simulink model "RefModel_FlightPerf"  (R2020a)
settings: Solver=ode1  StartTime=0.0  StopTime=10.0  FixedStep=Ts_Task.Ts_base  RelTol=1e-3
values from neighbouring files (symbols this model uses):
  TaskParam = TASK_SET.PathPlanner    [INIT_TASK.m]
undefined symbols (not defined in the file or in its folder): FlightPerfParam
settings Model: Creator=sl  LastModifiedBy=sl
settings DataIOCC: SaveOutput=off  SaveTime=off
settings OptimizationCC: DefaultParameterBehavior=Inlined  EnhancedBackFolding=on  PassReuseOutputArgsAs=Individual arguments  ZeroExternalMemoryAtStartup=off  ZeroInternalMemoryAtStartup=off  OptimizeBlockOrder=speed  DifferentSizesBufferReuse=on  OptimizationCustomize=off  EfficientTunableParamExpr=on
settings DebuggingCC: InheritedTsInSrcMsg=none  ParameterPrecisionLossMsg=none  ParameterTunabilityLossMsg=error  UnconnectedInputMsg=none  UnconnectedOutputMsg=none  UnconnectedLineMsg=none
settings HardwareCC: ProdBitPerPointer=32  ProdBitPerSizeT=32  ProdBitPerPtrDiffT=32  ProdLargestAtomicInteger=Long  ProdLargestAtomicFloat=Double  ProdWordSize=32  ProdHWDeviceType=ARM Compatible->ARM Cortex
settings ModelReferenceCC: ModelReferenceNumInstancesAllowed=Single  PropagateVarSize=During execution
settings SFSimCC: MATLABDynamicMemAlloc=off
settings RTWCC: SystemTargetFile=ert.tlc  TemplateMakefile=ert_default_tmf  GenerateReport=on  IncludeHyperlinkInReport=on  LaunchReport=on  GenerateTraceInfo=on  GenerateTraceReport=on  GenerateTraceReportSl=on  GenerateTraceReportSf=on  GenerateTraceReportEml=on
settings CodeAppCC: ForceParamTrailComments=on  IgnoreCustomStorageClasses=off  MaxIdLength=48  OperatorAnnotations=on  SimulinkDataObjDesc=on  SFDataObjDesc=on  MATLABFcnDesc=on  InsertBlockDesc=on  StateflowObjectComments=on  MATLABSourceComments=on
settings ERTTargetCC: TargetLangStandard=C99 (ISO)  GenerateSampleERTMain=on  LogVarNameModifier=none  SupportVariableSizeSignals=on  InlinedParameterPlacement=NonHierarchical  ERTCustomFileTemplate=example_file_process.tlc

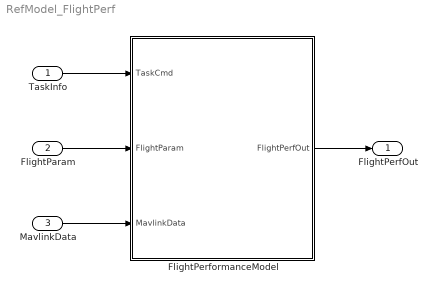
== system RefModel_FlightPerf ==
  TaskInfo : Inport  OutDataTypeStr=Bus: BUS_TASK_PATH_OutParam  BusOutputAsStruct=on
  FlightParam : Inport  Port=2  OutDataTypeStr=Bus: BUS_TASK_COMMON_OutParam  BusOutputAsStruct=on
  MavlinkData : Inport  Port=3  OutDataTypeStr=Bus: BUS_MAVLINK_TO_FIRM  PortDimensions=1  BusOutputAsStruct=on
  FlightPerformanceModel : Subsystem
  FlightPerfOut : Outport  OutDataTypeStr=Bus: BUS_FLIGHTPERF_OUT
  wires:
  MavlinkData/1 -> FlightPerformanceModel/3(MavlinkData)
  FlightPerformanceModel/1(FlightPerfOut) -> FlightPerfOut/1
  FlightParam/1 -> FlightPerformanceModel/2(FlightParam)
  TaskInfo/1 -> FlightPerformanceModel/1(TaskCmd)

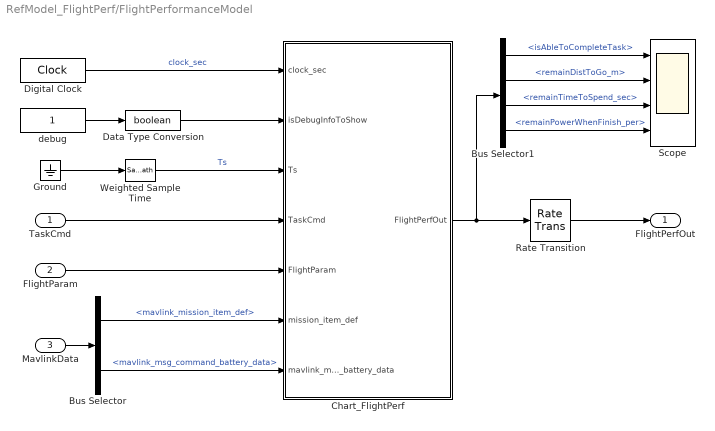
== system RefModel_FlightPerf/FlightPerformanceModel ==
  TaskCmd : Inport
  FlightParam : Inport  Port=2
  MavlinkData : Inport  Port=3
  Bus Selector : BusSelector  OutputSignals=mavlink_mission_item_def,mavlink_msg_command_battery_data
  Bus Selector1 : BusSelector  OutputSignals=isAbleToCompleteTask,remainDistToGo_m,remainTimeToSpend_sec,remainPowerWhenFinish_per
  Chart_FlightPerf : Stateflow chart  TreatAsAtomicUnit=on
  Data Type Conversion : DataTypeConversion  OutDataTypeStr=boolean
  Digital Clock : DigitalClock  SampleTime=-1
  Ground : Ground
  Rate Transition : RateTransition
  Scope : Scope  NumInputPorts=4
  Weighted Sample Time : SampleTimeMath  TsampMathOp=Ts Only
  debug : Constant
  FlightPerfOut : Outport
  wires:
  FlightParam/1 -> Chart_FlightPerf/5(FlightParam)
  debug/1 -> Data Type Conversion/1
  Data Type Conversion/1 -> Chart_FlightPerf/2(isDebugInfoToShow)
  Weighted Sample Time/1 -> Chart_FlightPerf/3(Ts)  "Ts"
  Digital Clock/1 -> Chart_FlightPerf/1(clock_sec)  "clock_sec"
  TaskCmd/1 -> Chart_FlightPerf/4(TaskCmd)
  MavlinkData/1 -> Bus Selector/1
  Ground/1 -> Weighted Sample Time/1
  Bus Selector/1 -> Chart_FlightPerf/6(mission_item_def)  "<mavlink_mission_item_def>"
  Chart_FlightPerf/1(FlightPerfOut) -> Bus Selector1/1, Rate Transition/1
  Bus Selector1/1 -> Scope/1  "<isAbleToCompleteTask>"
  Bus Selector1/2 -> Scope/2  "<remainDistToGo_m>"
  Bus Selector1/3 -> Scope/3  "<remainTimeToSpend_sec>"
  Bus Selector1/4 -> Scope/4  "<remainPowerWhenFinish_per>"
  Bus Selector/2 -> Chart_FlightPerf/7(mavlink_msg_command_battery_data)  "<mavlink_msg_command_battery_data>"
  Rate Transition/1 -> FlightPerfOut/1

== stateflow chart RefModel_FlightPerf/FlightPerformanceModel/Chart_FlightPerf ==
  state PowerConsumeByUavMode [parallel]
    settings: executionOrder=2
    state Rotor
      en:
    state Fix
      en:
    (default) -> PowerConsumeByUavMode.Rotor
    PowerConsumeByUavMode.Rotor -> Fix : [isUavInFix]
    Fix -> PowerConsumeByUavMode.Rotor : [isUavInRotor]
  state OverAllParam [parallel]
    settings: executionOrder=1
    state Rotor
      en:
      initFlightPerOut;
      du:
      on every(3,tick):
      predictDistToFly;
      on every(ceil(0.9/Ts),tick):
      predictTimeToFly;
      predictRemainPowerWhenComplete;
      isPowerEnoughToCompleteTask;
    (default) -> OverAllParam.Rotor
  data: flag function_output; debugInfo function_input; tabspace function_input; varargin function_input; flag function_output; modeName function_input; debugInfo function_input; varargin function_input; lla function_input; ll0 function_input; p function_output; clock_sec input; isDebugInfoToShow input; Ts input; TaskCmd input Bus: BUS_TASK_PATH_OutParam size=1; FlightParam input Bus: BUS_TASK_COMMON_OutParam size=1; mission_item_def input Bus: mavlink_mission_item_def size=TASK_SET.PathPlanner.maxPathPointNum; TaskParam parameter Bus: BUS_TASK_PATH_AlgoParam; FlightPerfParam parameter Bus: BUS_FLIGHTPERF_PARAM size=1; FlightPerfOut output Bus: BUS_FLIGHTPERF_OUT size=1; mavlink_msg_command_battery_data input Bus: mavlink_msg_command_battery_data size=1
  function predictRemainPowerWhenComplete:
    | function predictRemainPowerWhenComplete
    | persistent prePowerSpend hasEnterLandMode
    | if isempty(prePowerSpend)
    |     prePowerSpend = 0;
    |     hasEnterLandMode = false;
    | end
    | if FlightPerfOut.remainDistToGo_m == 0
    |     FlightPerfOut.remainTimeToSpend_sec = 0;
    |     return;
    | end
    | powerSpend = 0;
    | % 默认一个切换高度，对结果影响不大
    | switchHeight = 100;
    | curHeight = FlightParam.curLLA(3);
    | % 航线高度
    | pathHeight = double(mission_item_def(2).z);
    | % 模式耗时
    | powerSpend_TakeOff = 5;
    | powerSpend_HoverAfterTakeOff = 1;
    | powerSpend_Rotor2Fix = 0.2;
    | powerSpend_HoverUp = FlightPerfParam.powerRate_FixCruise*abs(pathHeight-switchHeight)/(TaskParam.maxClimbSpeed_fixMode+eps);
    | powerSpend_Path = FlightPerfParam.powerRate_FixCruise*FlightPerfOut.remainDistToGo_m/(TaskParam.cruiseSpeed_cruise+eps);
    | powerSpend_HoverDown = FlightPerfParam.powerRate_FixCruise*powerSpend_HoverUp;
    | powerSpend_Fix2Rotor = 0.5;
    | powerSpend_Land = 5;
    | if TaskCmd.flightTaskMode == ENUM_FlightTaskMode.LandMode
    |     hasEnterLandMode = true;
    | end
    | switch TaskCmd.flightTaskMode
    |     case ENUM_FlightTaskMode.GroundStandByMode
    |         if hasEnterLandMode
    |             powerSpend = 0;
    |         else
    |             powerSpend = ...
    |                 powerSpend_TakeOff + ...
    |                 powerSpend_HoverAfterTakeOff + ...
    |                 powerSpend_Rotor2Fix + ...
    |                 powerSpend_HoverUp + ...
    |                 powerSpend_Path + ...
    |                 powerSpend_HoverDown + ...
    |                 powerSpend_Fix2Rotor + ...
    |                 powerSpend_Land;
    |         end
    |     case ENUM_FlightTaskMode.TakeOffMode
    |         powerSpend = ...
    |             powerSpend_Rotor2Fix + ...
    |             powerSpend_HoverUp + ...
    |             powerSpend_Path + ...
    |             powerSpend_HoverDown + ...
    |             powerSpend_Fix2Rotor + ...
    |             powerSpend_Land;
    |         powerByThisTask = FlightPerfParam.powerRate_RotorNoWind*max(0,switchHeight-curHeight)/(TaskParam.maxClimbSpeed_normal_TakeOffandLand+eps);
    |         powerSpend = powerSpend + powerByThisTask;
    |     case ENUM_FlightTaskMode.HoverUpMode
    |         powerSpend = ...
    |             powerSpend_Path + ...
    |             powerSpend_HoverDown + ...
    |             powerSpend_Fix2Rotor + ...
    |             powerSpend_Land;
    |         powerByThisTask = FlightPerfParam.powerRate_FixCruise* max(0,pathHeight-curHeight)/(TaskParam.maxClimbSpeed_fixMode+eps);
    |         powerSpend = powerSpend + powerByThisTask;
    |     case ENUM_FlightTaskMode.PathFollowMode
    |         powerSpend = ...
    |             powerSpend_Path + ...
    |             powerSpend_HoverDown + ...
    |             powerSpend_Fix2Rotor + ...
    |             powerSpend_Land;
    |     case ENUM_FlightTaskMode.GoHomeMode
    |         powerSpend = ...
    |             powerSpend_Path + ...
    |             powerSpend_HoverDown + ...
    |             powerSpend_Fix2Rotor + ...
    |             powerSpend_Land;
    |     case ENUM_FlightTaskMode.HoverDownMode
    |         powerSpend = ...
    |             powerSpend_Fix2Rotor + ...
    |             powerSpend_Land;
    |         powerByThisTask = FlightPerfParam.powerRate_FixCruise*abs(curHeight-switchHeight)/(TaskParam.maxClimbSpeed_fixMode+eps);
    |         powerSpend = powerSpend + powerByThisTask;
    |     case ENUM_FlightTaskMode.LandMode
    |         powerSpend = 0.9*FlightPerfParam.powerRate_RotorNoWind*max(curHeight,0);
    |     otherwise
    |         powerSpend = prePowerSpend;
    | end
    | prePowerSpend = powerSpend;
    | FlightPerfOut.remainPowerWhenFinish_per = double(mavlink_msg_command_battery_data.battery(1).lifePercent) - powerSpend;
  function predictDistToFly:
    | function predictDistToFly
    | persistent hasEnterGoHomeMode remainDistToGo_movsmooth
    | if isempty(hasEnterGoHomeMode)
    |     hasEnterGoHomeMode = false;
    |     remainDistToGo_movsmooth = 0;
    | end
    | if TaskCmd.validPathNum == 0
    |     FlightPerfOut.remainDistToGo_m = 0;
    |     return;
    | end
    | validNum = 0;
    | maxNum = length(mission_item_def);
    | % 当前目标航点
    | if TaskCmd.currentPointNum ~= 0 % 进入航线模式前
    |     idx = TaskCmd.currentPointNum;
    | else
    |     idx = 2;
    | end
    | curPathPoint = double([mission_item_def(idx).x,mission_item_def(idx).y, mission_item_def(idx).z]);
    | % 最后一个航点
    | idx = TaskCmd.validPathNum;
    | lastValidPathPoint = double([mission_item_def(idx).x,mission_item_def(idx).y, mission_item_def(idx).z]);
    | % home点
    | idx = 1;
    | homePoint = double([mission_item_def(idx).x,mission_item_def(idx).y, mission_item_def(idx).z]);
    | % 当前位置
    | curLLA = FlightParam.curLLA;
    | %
    | FlightPerfOut.remainDistToGo_m = 0;
    | 
    | if TaskCmd.flightTaskMode == ENUM_FlightTaskMode.GoHomeMode
    |     hasEnterGoHomeMode = true;
    | end
    | %
    | if ~hasEnterGoHomeMode
    |     if TaskCmd.currentPointNum > 2
    |         idxStart = TaskCmd.currentPointNum;
    |     else
    |         idxStart = 2;
    |     end
    |     for idx = idxStart:maxNum
    |         tempPrePathPoint = double([mission_item_def(idx).x,mission_item_def(idx).y, mission_item_def(idx).z]);
    |         tempCurPathPoint = double([mission_item_def(idx+1).x,mission_item_def(idx+1).y, mission_item_def(idx+1).z]);
    |         tempPos = lla2ned(tempPrePathPoint, tempCurPathPoint(1:2));
    |         tempDist = norm(tempPos);
    |         if idx <= TaskCmd.validPathNum-1 && isPathPointValid(curPathPoint)
    |             FlightPerfOut.remainDistToGo_m = FlightPerfOut.remainDistToGo_m + tempDist + FlightPerfParam.addedDistByEachTurnCorrect;
    |         else
    |             break;
    |         end
    |     end
    |     tempPos = lla2ned(curLLA, curPathPoint(1:2));
    |     distToCurPathPoint = norm(tempPos);
    |     tempPos = lla2ned(lastValidPathPoint, homePoint(1:2));
    |     distFromEndPointToHome = norm(tempPos);
    |     FlightPerfOut.remainDistToGo_m = FlightPerfOut.remainDistToGo_m + distToCurPathPoint + distFromEndPointToHome;
    | else
    |     tempPos = lla2ned(curLLA, homePoint(1:2));
    |     distFromCurLLAToHome = norm(tempPos);
    |     FlightPerfOut.remainDistToGo_m = distFromCurLLAToHome;
    | end
    | FlightPerfOut.remainDistToGo_m = movsmooth(FlightPerfOut.remainDistToGo_m);
    | end
    | %% 子函数
    | % 
    | function out = movsmooth(val)
    | persistent valsmooth
    | if isempty(valsmooth)
    |     valsmooth = 0;
    | end
    | if val ~= 0
    | %     if norm(valsmooth-val)<2000
    |         kscale = 11/12;
    |         valsmooth = kscale*valsmooth + (1-kscale)*val;
    |         out = valsmooth;
    | %     else
    | %         out = val;
    | %     end
    | else
    |     out = 0;
    | end
    | end
    | % 
    | function flag = isPathPointValid(LLA)
    | flag = true;
    | for i_LLA = 1:2
    |     if abs(LLA(i_LLA)) > 360
    |         flag = false;
    |     end
    | end
    | end
  function flag = isUavInRotor:
    | function flag = isUavInRotor
    | flag = false;
    | if TaskCmd.uavMode == ENUM_UAVMode.Rotor
    |     flag = true;
    | end
  function printComInfo(debugInfo,tabspace,varargin):
    | function printComInfo(debugInfo,tabspace,varargin)
    | if nargin == 3
    |     value = double(varargin{1});
    |     noValue = false;
    | else
    |     value = 0;
    |     noValue = true;
    | end
    | if isDebugInfoToShow
    |     if ~noValue
    |         switch tabspace
    |             case 0
    |                 fprintf([' %.3f sec: ',debugInfo,'\n'],clock_sec,value);
    |             case 1
    |                 fprintf(['\t %.3f sec: ',debugInfo,'\n'],clock_sec,value);
    |             case 2
    |                 fprintf(['\t\t %.3f sec: ',debugInfo,'\n'],clock_sec,value);
    |             case 3
    |                 fprintf(['\t\t\t %.3f sec: ',debugInfo,'\n'],clock_sec,value);
    |             case 4
    |                 fprintf(['\t\t\t\t %.3f sec: ',debugInfo,'\n'],clock_sec,value);
    |         end
    |     else
    |         switch tabspace
    |             case 0
    |                 fprintf([' %.3f sec: ',debugInfo,'\n'],clock_sec);
    |             case 1
    |                 fprintf(['\t %.3f sec: ',debugInfo,'\n'],clock_sec);
    |             case 2
    |                 fprintf(['\t\t %.3f sec: ',debugInfo,'\n'],clock_sec);
    |             case 3
    |                 fprintf(['\t\t\t %.3f sec: ',debugInfo,'\n'],clock_sec);
    |             case 4
    |                 fprintf(['\t\t\t\t %.3f sec: ',debugInfo,'\n'],clock_sec);
    |         end        
    |     end
    | end
  function isPowerEnoughToCompleteTask:
    | function isPowerEnoughToCompleteTask
    | if FlightPerfOut.remainPowerWhenFinish_per < TaskParam.low_battery_alarm_set
    |     FlightPerfOut.isAbleToCompleteTask = false;
    | else 
    |     FlightPerfOut.isAbleToCompleteTask = true;
    | end
  function predictTimeToFly:
    | function predictTimeToFly
    | persistent preTimeSpend hasEnterLandMode
    | if isempty(preTimeSpend)
    |     preTimeSpend = 0;
    |     hasEnterLandMode = false;
    | end
    | if FlightPerfOut.remainDistToGo_m == 0
    |     FlightPerfOut.remainTimeToSpend_sec = 0;
    |     return;
    | end
    | timeSpend = 0;
    | % 默认一个切换高度，对结果影响不大
    | switchHeight = 100;
    | curHeight = FlightParam.curLLA(3);
    | % 航线高度
    | pathHeight = double(mission_item_def(2).z);
    | % 模式耗时
    | timeSpend_TakeOff = 10 + switchHeight/(TaskParam.maxClimbSpeed_normal_TakeOffandLand+eps);
    | timeSpend_HoverAfterTakeOff = 10;
    | timeSpend_Rotor2Fix = 10;
    | timeSpend_HoverUp = abs(pathHeight-switchHeight)/(TaskParam.maxClimbSpeed_fixMode+eps);
    | timeSpend_Path = FlightPerfOut.remainDistToGo_m/(TaskParam.cruiseSpeed_cruise+eps);
    | timeSpend_HoverDown = timeSpend_HoverUp;
    | timeSpend_Fix2Rotor = 10;
    | timeSpend_Land = timeSpend_TakeOff;
    | if TaskCmd.flightTaskMode == ENUM_FlightTaskMode.LandMode
    |     hasEnterLandMode = true;
    | end
    | switch TaskCmd.flightTaskMode
    |     case ENUM_FlightTaskMode.GroundStandByMode
    |         if hasEnterLandMode
    |             timeSpend = 0;
    |         else
    |             timeSpend = ...
    |                 timeSpend_TakeOff + ...
    |                 timeSpend_HoverAfterTakeOff + ...
    |                 timeSpend_Rotor2Fix + ...
    |                 timeSpend_HoverUp + ...
    |                 timeSpend_Path + ...
    |                 timeSpend_HoverDown + ...
    |                 timeSpend_Fix2Rotor + ...
    |                 timeSpend_Land;
    |         end
    |     case ENUM_FlightTaskMode.TakeOffMode
    |         timeSpend = ...
    |             timeSpend_Rotor2Fix + ...
    |             timeSpend_HoverUp + ...
    |             timeSpend_Path + ...
    |             timeSpend_HoverDown + ...
    |             timeSpend_Fix2Rotor + ...
    |             timeSpend_Land;
    |         timeByThisTask = 10 + max(0,switchHeight-curHeight)/(TaskParam.maxClimbSpeed_normal_TakeOffandLand+eps);
    |         timeSpend = timeSpend + timeByThisTask;
    |     case ENUM_FlightTaskMode.HoverUpMode
    |         timeSpend = ...
    |             timeSpend_Path + ...
    |             timeSpend_HoverDown + ...
    |             timeSpend_Fix2Rotor + ...
    |             timeSpend_Land;
    |         timeByThisTask = 10 + max(0,pathHeight-curHeight)/(TaskParam.maxClimbSpeed_fixMode+eps);
    |         timeSpend = timeSpend + timeByThisTask;
    |     case ENUM_FlightTaskMode.PathFollowMode
    |         timeSpend = ...
    |             timeSpend_Path + ...
    |             timeSpend_HoverDown + ...
    |             timeSpend_Fix2Rotor + ...
    |             timeSpend_Land;
    |     case ENUM_FlightTaskMode.GoHomeMode
    |         timeSpend = ...
    |             timeSpend_Path + ...
    |             timeSpend_HoverDown + ...
    |             timeSpend_Fix2Rotor + ...
    |             timeSpend_Land;
    |     case ENUM_FlightTaskMode.HoverDownMode
    |         timeSpend = ...
    |             timeSpend_Fix2Rotor + ...
    |             timeSpend_Land;
    |         timeByThisTask = abs(curHeight-switchHeight)/(TaskParam.maxClimbSpeed_fixMode+eps);
    |         timeSpend = timeSpend + timeByThisTask;
    |     case ENUM_FlightTaskMode.LandMode
    |         timeSpend = max(curHeight,0);
    |     otherwise
    |         timeSpend = preTimeSpend;
    | end
    | preTimeSpend = double(timeSpend);
    | FlightPerfOut.remainTimeToSpend_sec = double(timeSpend);
    | 
    | %% 子函数
  function flag = isUavInFix:
    | function flag = isUavInFix
    | flag = false;
    | if TaskCmd.uavMode == ENUM_UAVMode.Fix
    |     flag = true;
    | end
  function printDebugInfo(modeName,debugInfo,varargin):
    | function printDebugInfo(modeName,debugInfo,varargin)
    | if nargin == 3
    |     tabspace = varargin{1};
    | else
    |     tabspace = 2;
    | end
    | if isDebugInfoToShow
    |     switch tabspace
    |         case 0
    |             fprintf(' %.3f sec: [%s] %s\n',clock_sec,modeName,debugInfo);
    |         case 1
    |             fprintf('\t %.3f sec: [%s] %s\n',clock_sec,modeName,debugInfo);
    |         case 2
    |             fprintf('\t\t %.3f sec: [%s] %s\n',clock_sec,modeName,debugInfo);
    |         case 3
    |             fprintf('\t\t\t %.3f sec: [%s] %s\n',clock_sec,modeName,debugInfo);
    |         case 4
    |             fprintf('\t\t\t\t %.3f sec: [%s] %s\n',clock_sec,modeName,debugInfo);
    |     end
    | end
  function p = lla2ned(lla, ll0):
    | function p = lla2ned(lla, ll0)
    | % 纬经高转换为NED位置
    | % lla: 纬度[deg] 经度[deg] 高度[m] 
    | % ll0: 基准点， 纬度[deg] 经度[deg]
    | % p: NED位置
    | p = zeros(1,3);
    | psi0 = 0;
    | href = 0;
    | f = 0.003352810664747;
    | R = 6378.137e3;
    | % wrap latitude and longitude if needed
    | [~, lla(:,1), lla(:,2)] = wraplatitude( lla(:,1), lla(:,2), 'deg' );
    | [~, ll0(1), ll0(2)] = wraplatitude( ll0(1), ll0(2), 'deg' );
    | 
    | % check and fix angle wrapping in longitude
    | [~, lla(:,2)] = wraplongitude( lla(:,2), 'deg', '180' );
    | [~, ll0(2)] = wraplongitude( ll0(2), 'deg', '180' );
    | 
    | dLat = lla(:,1) - ll0(1);
    | dLon = lla(:,2) - ll0(2);
    | 
    | % wrap latitude and longitude if needed
    | [~, dLat, dLon] = wraplatitude( dLat', dLon', 'deg' );
    | 
    | % check and fix angle wrapping in longitude
    | [~, dLon] = wraplongitude( dLon, 'deg', '180' );
    | 
    | rll0 = ll0*pi/180;
    | rpsi0 = psi0*pi/180;
    | 
    | Rn = R/sqrt(1-(2*f-f*f)*sin(rll0(1))*sin(rll0(1)));
    | Rm = Rn*((1-(2*f-f*f))/(1-(2*f-f*f)*sin(rll0(1))*sin(rll0(1))));
    | 
    | dNorth = dLat./atan2(1,Rm)*pi/180;
    | dEast = dLon./atan2(1,Rn*cos(rll0(1)))*pi/180;
    | 
    | p(:,1) = cos(rpsi0)*dNorth + sin(rpsi0)*dEast;
    | p(:,2) = -sin(rpsi0)*dNorth + cos(rpsi0)*dEast;
    | p(:,3) = -lla(:,3) - href;
    | end
    | 
    | function [lat_wrapped, lat, lon] = wraplatitude( lat, lon, units)
    | % WRAPLATITUDE internal function to check and fix angle wrapping in
    | % latitude and longitude if needed.
    | 
    | %   Copyright 2007-2013 The MathWorks, Inc.
    | 
    | % Convert units if necessary
    | if strcmp(units,'deg')
    |     pideg = 180;
    | else
    |     pideg = pi;
    | end
    | 
    | % Set lat_wrapped flag to false
    | lat_wrapped = false;
    | 
    | % Re-set latitudes to values between pi and -pi
    | flat = abs(lat);
    | 
    | if any(flat>pideg)
    |     lat(flat>pideg) = mod(lat(flat>pideg)+pideg,2*pideg)-pideg;
    |     % Set lat_wrapped flag to true if necessary
    |     flat = abs(lat);
    |     lat_wrapped = true;
    | end
    | 
    | % Determine if any latitudes need to be wrapped
    | idx = flat>pideg/2;
    | 
    | if any(idx)
    |     
    |     % Adjustments for -pi to pi
    |     flat = abs(lat);
    |     latp2 = flat>pideg/2;
    |     lon(idx) = lon(idx) + pideg;
    |     lat(latp2) = sign(lat(latp2)).*(pideg/2-(flat(latp2)-pideg/2));
    |     
    |     % Set lat_wrapped flag to true if necessary
    |     lat_wrapped = true;
    |     
    | end
    | end
    | 
    | function [lon_wrapped, lon] = wraplongitude( lon, inputUnits, maxRange )
    | % WRAPLONGITUDE internal function to check and fix angle wrapping in
    | % longitude.
    | 
    | %   Copyright 2007-2010 The MathWorks, Inc.
    | 
    | % Convert units if necessary
    | if strcmp(inputUnits,'deg')
    |     lon = lon*pi/180;
    | end
    | 
    | lon_wrapped = false;
    | 
    | switch maxRange
    |     % Range goes between -pi and pi
    |     case {'180','pi'}
    |         idx = lon > pi | lon < -pi;
    |         if any(idx)
    |             lon(idx) = rem(lon(idx),2*pi)- (2*pi)*fix(rem(lon(idx),2*pi)/pi);
    |             lon_wrapped = true;
    |         end
    |     % Range goes between 0 and 2*pi
    |     case {'360','2*pi'}
    |         idx = lon > 2*pi | lon < 0;
    |         if any(idx)
    |             lon(idx) = mod(lon(idx),2*pi);
    |             lon_wrapped = true;
    |         end
    |     otherwise
    |         % do nothing
    | end
    | 
    | % Convert units if necessary
    | if strcmp(inputUnits,'deg')
    |     lon = lon*180/pi;
    | end
    | end
  function initFlightPerOut:
    | function initFlightPerOut
    | FlightPerfOut.isAbleToCompleteTask = true;
    | FlightPerfOut.remainDistToGo_m = 0;
    | FlightPerfOut.remainTimeToSpend_sec = 0;
    | FlightPerfOut.remainPowerWhenFinish_per = 0;
